simulink model "freqsyn"  (Simulink 6.0)
settings: Solver=ode45  StartTime=0.0  StopTime=500*synM/synFr  FixedStep=1/(3*synFr*synN/synM)  MaxStep=.5/(synFr*synN/synM)  RelTol=1e-3
PreLoadFcn:
  | synM = 3;    % frequency division ratio
  | synN = 10;   % frequency division ratio
  | synFr = 30e6;   % reference frequency
  | synFq = synFr;       % quiescent frequency
  | synSen = 40e6;   % VCO sensitivity
model workspace: external: M-Code (data not in the file)
undefined symbols (not defined in the file or in its folder): slcm
libraries: commblksprivate x2, dsparch4 x1, commsynccomp2 x1
CloseFcn:
  | clear synM synN synFr synFq synSen synSigsOut
settings Model: CovMetricSettings=d  Creator=ysong  LastModifiedBy=fwei  ExtModeAutoUpdateStatusClock=off
settings DataIOCC: SaveOutput=off  SaveTime=off  SignalLoggingName=synSigsOut
settings OptimizationCC: BlockReduction=off  BooleanDataType=off
settings DebuggingCC: CheckExecutionContextPreStartOutputMsg=on  CheckExecutionContextRuntimeOutputMsg=on  SolverPrmCheckMsg=none
settings HardwareCC: TargetUnknown=on
settings ModelReferenceCC: UpdateModelReferenceTargets=IfOutOfDate
settings GRTTargetCC: LifeSpan=inf
settings SFSimCC: SFSimApplyToAllLibs=on  SFSimBuildMode=Incremental

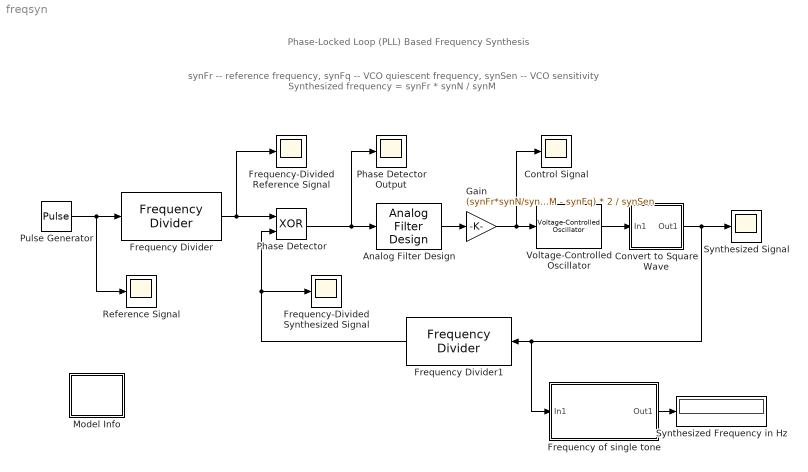
== system freqsyn ==
  note: Phase-Locked Loop (PLL) Based Frequency Synthesis
  note: synFr -- reference frequency,  synFq -- VCO quiescent frequency,  synSen -- VCO sensitivity
      | Synthesized frequency = synFr * synN / synM
  Analog Filter Design : dsparch4/Analog Filter Design  method=Butterworth  filttype=Lowpass  N=1  Wlo=synFr/synM/10  Whi=80  Rp=2  Rs=40
  Control Signal : Scope
      settings: TimeRange=5e-005  YMin=0  YMax=2.5
  Convert to Square Wave : Subsystem  EnableExecutionContextPropagation=on
  Frequency Divider : commblksprivate/Frequency Divider  n=synM
  Frequency Divider1 : commblksprivate/Frequency Divider  Orientation=left  n=synN
  Frequency of single tone : Subsystem  EnableExecutionContextPropagation=on
      mask Display: disp('Single Tone\nFrequency Estimator');
  Frequency-Divided Reference Signal : Scope
      settings: TimeRange=2e-007  YMin=-1  YMax=2  SaveName=ScopeData5
  Frequency-Divided Synthesized Signal : Scope
      settings: TimeRange=2e-007  YMin=-1  YMax=2  SaveName=ScopeData4
  Gain : Gain  Gain=(synFr*synN/synM - synFq) * 2 / synSen  SaturateOnIntegerOverflow=on
  Model Info : Subsystem  LoadFcn=slcm LoadBlock;  InitFcn=slcm('UpdateAllCMBlocksInThisModelInit')  EnableExecutionContextPropagation=on  mask(CMBlock){InitialSaveTempField=, InitialBlockCM=none, BlockCM=none, Frame=on, SaveTempField=, DisplayStringWithTags=Info, MaskDisplayString=Info, HorizontalTextAlignment=Center, LeftAlignmentValue=0.5, SourceBlockDiagram=freqsyn, TagMaxNumber=20, CMTag1=, CMTag2=, CMTag3=, CMTag4=, CMTag5=, CMTag6=, CMTag7=, CMTag8=, CMTag9=, CMTag10=, CMTag11=, CMTag12=, CMTag13=, CMTag14=, CMTag15=, CMTag16=, CMTag17=, CMTag18=, CMTag19=, CMTag20=}
      mask help: This block allows revision control information to be displayed within the model.
      settings: CopyFcn=slcm CopyBlock;  DeleteFcn=slcm Cancel;  PostSaveFcn=slcm('UpdateAllCMBlocksInThisModel')  NameChangeFcn=slcm Rename;  OpenFcn=commdemohelp;
      mask Display: text(str2num(LeftAlignmentValue), 0.5, MaskDisplayString, 'HorizontalAlignment', HorizontalTextAlignment)
  Phase Detector : Logic  Operator=XOR
  Phase Detector Output : Scope
      settings: TimeRange=2e-007  YMin=-1  YMax=2  SaveName=ScopeData6
  Pulse Generator : DiscretePulseGenerator  PulseType=Time based  Period=1/synFr  PulseWidth=50
  Reference Signal : Scope
      settings: TimeRange=1e-007  YMin=-1  YMax=2
  Synthesized Signal : Scope
      settings: TimeRange=5e-008  YMin=-1  YMax=2  SaveName=ScopeData2  MaxDataPoints=50000
  Synthesized Frequency in Hz : Display
  Voltage-Controlled Oscillator : commsynccomp2/Voltage-Controlled Oscillator  Ac=1  Fc=synFq  Kc=synSen  Ph=0
  wires:
  Pulse Generator/1 -> Reference Signal/1, Frequency Divider/1
  Phase Detector/1 -> Analog Filter Design/1, Phase Detector Output/1
  Gain/1 -> Voltage-Controlled Oscillator/1, Control Signal/1
  Voltage-Controlled Oscillator/1 -> Convert to Square Wave/1(In1)
  Convert to Square Wave/1(Out1) -> Synthesized Signal/1, Frequency Divider1/1, Frequency of single tone/1(In1)
  Frequency Divider/1 -> Phase Detector/1, Frequency-Divided Reference Signal/1
  Frequency Divider1/1 -> Phase Detector/2, Frequency-Divided Synthesized Signal/1
  Analog Filter Design/1 -> Gain/1
  Frequency of single tone/1(Out1) -> Synthesized Frequency in Hz/1

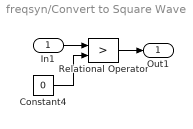
== system freqsyn/Convert to Square Wave ==
  In1 : Inport  LatchInput=off
  Constant4 : Constant  Value=0
  Relational Operator : RelationalOperator  Operator=>  InputSameDT=on
  Out1 : Outport
  wires:
  Relational Operator/1 -> Out1/1
  In1/1 -> Relational Operator/1
  Constant4/1 -> Relational Operator/2

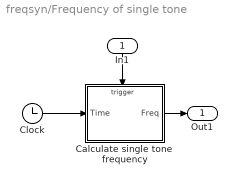
== system freqsyn/Frequency of single tone ==
  In1 : Inport  Orientation=down  LatchInput=off
  Calculate single tone  frequency : Subsystem  TreatAsAtomicUnit=on  EnableExecutionContextPropagation=on
  Clock : Clock
  Out1 : Outport
  wires:
  Calculate single tone  frequency/1(Freq) -> Out1/1
  Clock/1 -> Calculate single tone  frequency/1(Time)
  In1/1 -> Calculate single tone  frequency/Trigger

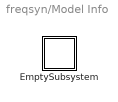
== system freqsyn/Model Info ==
  EmptySubsystem : Subsystem  EnableExecutionContextPropagation=on

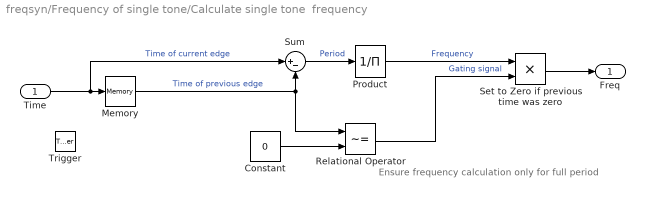
== system freqsyn/Frequency of single tone/Calculate single tone  frequency ==
  note: Ensure frequency calculation
      | only for full period
  Time : Inport  LatchInput=off
  Trigger : TriggerPort  ZeroCross=off
  Constant : Constant  Value=0
  Memory : Memory  InheritSampleTime=on
  Product : Product  Inputs=/  SaturateOnIntegerOverflow=on  InputSameDT=on
  Relational Operator : RelationalOperator  Operator=~=  InputSameDT=on
  Set to Zero if previous time was zero : Product  SaturateOnIntegerOverflow=on  InputSameDT=on
  Sum : Sum  Inputs=|+-  SaturateOnIntegerOverflow=on  InputSameDT=on
  Freq : Outport  InitialOutput=0
  wires:
  Relational Operator/1 -> Set to Zero if previous time was zero/2  "Gating signal"
  Constant/1 -> Relational Operator/2
  Set to Zero if previous time was zero/1 -> Freq/1
  Memory/1 -> Relational Operator/1, Sum/2  "Time of previous edge"
  Product/1 -> Set to Zero if previous time was zero/1  "Frequency"
  Sum/1 -> Product/1  "Period"
  Time/1 -> Memory/1, Sum/1  "Time of current edge"

== system freqsyn/Model Info/EmptySubsystem ==
